simulink model "PD_gravity"  (R2024b)
settings: Solver=ode3  StartTime=0.0  StopTime=inf  FixedStep=0.001  RelTol=1e-3
values from neighbouring files (symbols this model uses):
  p = zeros(60,1)    [UR5e_init.m]
  q0 = zeros(6,1)    [UR5e_init.m]
libraries: robotsim3dlib x1, sim3dlib x1
settings Model: Creator=feder  LastModifiedBy=feder

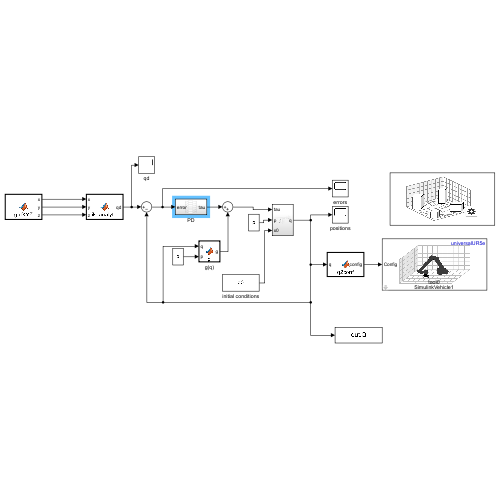
[thumbnail: Simulink's stored preview of the top-level diagram]
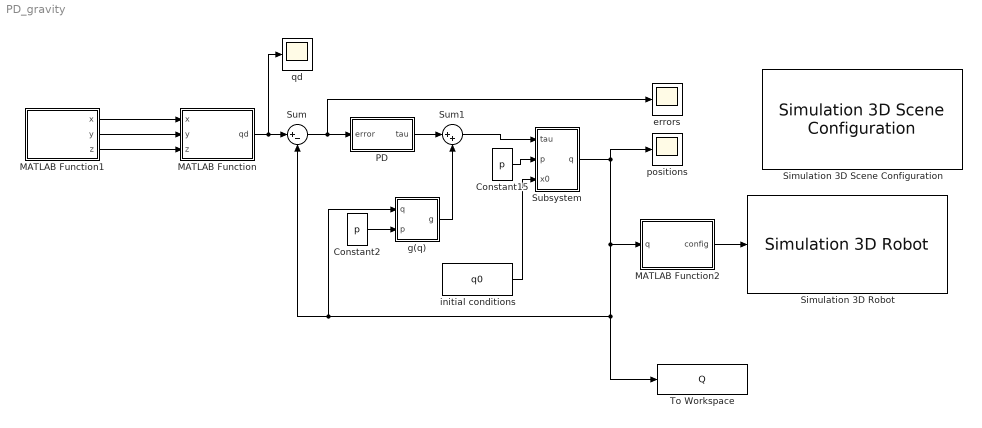
== system PD_gravity ==
  Constant15 : Constant  Value=p
  Constant2 : Constant  Value=p
  MATLAB Function : MATLAB Function  TreatAsAtomicUnit=on
  MATLAB Function1 : MATLAB Function  TreatAsAtomicUnit=on
  MATLAB Function2 : MATLAB Function  TreatAsAtomicUnit=on
  PD : Subsystem
  Simulation 3D Robot : robotsim3dlib/Simulation 3D Robot  actorInputType=Robot Library  RigidBodyTree=universalUR5e  ActorName=SimulinkVehicle1  existActorChekBox=off  initialTrans=[0 0 0]  initialRot=[0 0 0]  initialConfig="[0  0  0  0  0  0]"  EndEffector=tool0  eeOffsetInpChekBox=off  eeTargetTrans=[0 0 0]  eeTargetRot=[0 0 0]  enableRegionGraspChekBox=off  regionGraspInpChekBox=off  eeTargTransDiff=[0.2 0.2 0.2]  eeTargRotDiff=[0 0 0]  inpConfEnbVal=on  inpGraspEnbVal=off  inpTransEnbVal=off  outConfEnbVal=off  outGraspEnbVal=off  outTransEnbVal=off  SampleTime=0.01  ActorType=SimulinkVehicle  ID=1  aMode=6  ActorTag=SimulinkVehicle1  Mesh=RigidBodyTree
  Simulation 3D Scene Configuration : sim3dlib/Simulation 3D Scene Configuration  Priority=0  ProjectFormat=Default Scenes  SceneDesc=Double lane change  ProjectName=C:\Program Files\MATLAB\R2024b\toolbox\shared\sim3d_projects\automotive_project_windows\UE\WindowsNoEditor\VehicleSimulation.exe  ScenePath=/Game/Maps/EmptyScene  EnableOpenDRIVE=off  vehTagList={'Custom';'Scene Origin';'SimulinkVehicle1'}  vehTag=Scene Origin  FreeCameraInitialTranslation=[0, 0, 0]  FreeCameraDefaultInitialTranslation=[-6, 0, 2]  FreeCameraInitialRotation=[0, 0, 0]  FreeCameraDefaultInitialRotation=[0, -15, 0]  OpVisEn=off  Ts=0.001  EnableWindow=on  EnableRemoteAccess=off  EnableWeather=off  SunAzimuth=90  SunAltitude=40.0  EnableGeospatialSun=off  Latitude=0  Longitude=0  Date=2023-01-01  Time=10:30:00  GeoTimeZone=-5.0  SunDaylightSaving=off  wind=1  clouds=10  EnableVolumetricClouds=off  CloudCoverage=0  CloudAltitude=6  fog=0  rain=0  RaindropsEffect=off  SnowDensity=0  EnableGeospatial=off  UseTrueOrigin=off  OriginHeight=200  OriginLatitude=40.744652  OriginLongitude=-73.988864  MapStyle=Aerial  AdditionalAssetIDs=[]  UseAdvancedSunSky=off  SolarTime=11  TimeZone=-5  Day=21  Month=9  Year=2022  UseDaylightSavingTime=on  DSTStartDay=10  DSTStartMonth=3  DSTEndDay=3  DSTEndMonth=11  DSTSwitchHour=2  sensorTag=MainCamera1  sensorId=1  sensorName=MainCamera1  mountLoc=Origin  offsetFlag=off  tmountOffset=[0, 0, 0]  rmountOffset=[0, 0, 0]  HorizontalResolution=1280  VerticalResolution=720  HorizontalFOV=60  mountPoint=[0 0 0]  mountOrientation=[0 0 0]  aMode=6  ID=1  GeoTrigger=Inactive
      settings: LibrarySourceBlock=robotsim3dlib/Simulation 3D Scene Configuration
  Subsystem : Subsystem
  Sum : Sum  Inputs=|+-
  Sum1 : Sum  Inputs=|++
  To Workspace : ToWorkspace  VariableName=Q  SampleTime=0.01
      settings: MaxDataPoints=10
  errors : Scope
  g(q) : MATLAB Function  TreatAsAtomicUnit=on
  initial conditions : Constant  Value=q0
  positions : Scope
  qd : Scope
  wires:
  Constant2/1 -> g(q)/2(p)
  Subsystem/1(q) -> MATLAB Function2/1(q), To Workspace/1, g(q)/1(q), Sum/2, positions/1
  Sum1/1 -> Subsystem/1(tau)
  MATLAB Function/1(qd) -> qd/1, Sum/1
  g(q)/1(g) -> Sum1/2
  initial conditions/1 -> Subsystem/3(x0)
  PD/1(tau) -> Sum1/1
  Constant15/1 -> Subsystem/2(p)
  Sum/1 -> errors/1, PD/1(error)
  MATLAB Function1/1(x) -> MATLAB Function/1(x)
  MATLAB Function1/3(z) -> MATLAB Function/3(z)
  MATLAB Function1/2(y) -> MATLAB Function/2(y)
  MATLAB Function2/1(config) -> Simulation 3D Robot/1

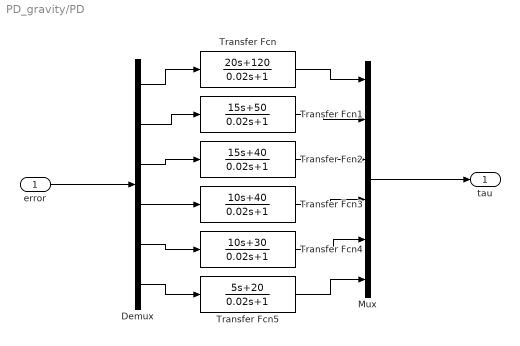
== system PD_gravity/PD ==
  error : Inport  PortDimensions=6
  Demux : Demux  Outputs=6
  Mux : Mux  Inputs=6
  Transfer Fcn : TransferFcn  Numerator=[20 120]  Denominator=[0.02 1]
  Transfer Fcn1 : TransferFcn  Numerator=[15 50]  Denominator=[0.02 1]
  Transfer Fcn2 : TransferFcn  Numerator=[15 40]  Denominator=[0.02 1]
  Transfer Fcn3 : TransferFcn  Numerator=[10 40]  Denominator=[0.02 1]
  Transfer Fcn4 : TransferFcn  Numerator=[10 30]  Denominator=[0.02 1]
  Transfer Fcn5 : TransferFcn  Numerator=[5 20]  Denominator=[0.02 1]
  tau : Outport  PortDimensions=6
  wires:
  Demux/1 -> Transfer Fcn/1
  Demux/2 -> Transfer Fcn1/1
  error/1 -> Demux/1
  Transfer Fcn/1 -> Mux/1
  Transfer Fcn1/1 -> Mux/2
  Mux/1 -> tau/1
  Demux/3 -> Transfer Fcn2/1
  Transfer Fcn2/1 -> Mux/3
  Demux/4 -> Transfer Fcn3/1
  Demux/5 -> Transfer Fcn4/1
  Demux/6 -> Transfer Fcn5/1
  Transfer Fcn3/1 -> Mux/4
  Transfer Fcn4/1 -> Mux/5
  Transfer Fcn5/1 -> Mux/6

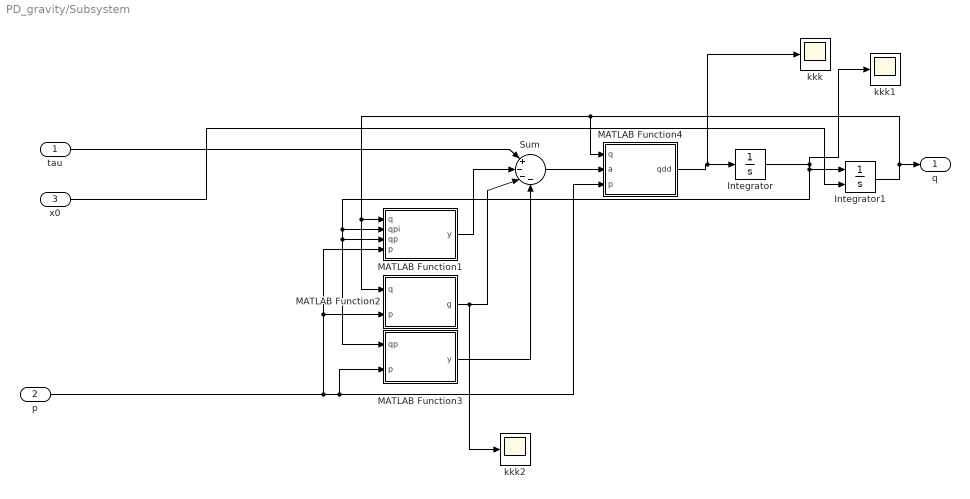
== system PD_gravity/Subsystem ==
  tau : Inport  PortDimensions=6
  p : Inport  Port=2
  x0 : Inport  Port=3
  Integrator : Integrator  InitialCondition=[0.1;0.1;0.1;0.1;0.1;0.1]
  Integrator1 : Integrator  InitialConditionSource=external
  MATLAB Function1 : MATLAB Function  TreatAsAtomicUnit=on
  MATLAB Function2 : MATLAB Function  TreatAsAtomicUnit=on
  MATLAB Function3 : MATLAB Function  TreatAsAtomicUnit=on
  MATLAB Function4 : MATLAB Function  TreatAsAtomicUnit=on
  Sum : Sum  Inputs=|+---
  kkk : Scope
  kkk1 : Scope
  kkk2 : Scope
  q : Outport  PortDimensions=6
  wires:
  MATLAB Function2/1(g) -> kkk2/1, Sum/3
  p/1 -> MATLAB Function1/4(p), MATLAB Function2/2(p), MATLAB Function3/2(p), MATLAB Function4/3(p)
  Integrator1/1 -> MATLAB Function2/1(q), MATLAB Function1/1(q), MATLAB Function4/1(q), q/1
  tau/1 -> Sum/1
  Sum/1 -> MATLAB Function4/2(a)
  Integrator/1 -> Integrator1/1, MATLAB Function1/3(qp), MATLAB Function3/1(qp), MATLAB Function1/2(qpi), kkk1/1
  MATLAB Function1/1(y) -> Sum/2
  MATLAB Function3/1(y) -> Sum/4
  x0/1 -> Integrator1/2
  MATLAB Function4/1(qdd) -> Integrator/1, kkk/1

== matlab function PD_gravity/Subsystem/MATLAB Function1 ==
  data: q input; qpi input; qp input; y output; p input
function y = Cqp(q, qpi, qp, p)
% Cqp_rt_full
% Approssimazione real-time safe di C(q,qd)*qd per UR5e
% Considera tutti gli accoppiamenti principali tra i 6 giunti e i bracci r_i
%
% Input:
% q   [6x1] : posizioni articolari
% qpi [6x1] : velocità articolari (alias di qp, per compatibilità)
% qp  [6x1] : velocità articolari
% p   [60x1]: parametri dinamici UR5e
%
% Output:
% y [6x1] : C(q,qd)*qd approssimato

y = zeros(6,1);

% % ----------------------------
% % Estrazione parametri principali
% % ----------------------------
% m = zeros(6,1);
% r = zeros(6,3);
% 
% for i = 1:6
%     idx = (i-1)*10;
%     m(i) = p(idx+1);            % massa
%     r(i,:) = p(idx+2:idx+4)';   % m*r già incluso in p
% end
% 
% % ----------------------------
% % Termini principali di Coriolis
% % Formula: c_ij = m_j * sin(q_j) * (r_j · r_effect) * qdot_i * qdot_j
% % ----------------------------
% 
% % Giunto 1-2
% y(1) = -m(2) * sin(q(2)) * dot(r(2,:), r(1,:)) * qp(2) * qp(1);
% y(2) =  m(2) * sin(q(2)) * dot(r(2,:), r(1,:)) * qp(1) * qp(2);
% 
% % Giunto 2-3
% y(2) = y(2) - m(3) * sin(q(3)) * dot(r(3,:), r(2,:)) * qp(3) * qp(2);
% y(3) =  m(3) * sin(q(3)) * dot(r(3,:), r(2,:)) * qp(2) * qp(3);
% 
% % Giunto 3-4
% y(3) = y(3) - m(4) * sin(q(4)) * dot(r(4,:), r(3,:)) * qp(4) * qp(3);
% y(4) =  m(4) * sin(q(4)) * dot(r(4,:), r(3,:)) * qp(3) * qp(4);
% 
% % Giunto 4-5
% y(4) = y(4) - m(5) * sin(q(5)) * dot(r(5,:), r(4,:)) * qp(5) * qp(4);
% y(5) =  m(5) * sin(q(5)) * dot(r(5,:), r(4,:)) * qp(4) * qp(5);
% 
% % Giunto 5-6
% y(5) = y(5) - m(6) * sin(q(6)) * dot(r(6,:), r(5,:)) * qp(6) * qp(5);
% y(6) =  m(6) * sin(q(6)) * dot(r(6,:), r(5,:)) * qp(5) * qp(6);

end

== matlab function PD_gravity/g(q) ==
  data: q input; g output; p input
function g = g(q, p)
% g_fullJacobian
% Calcola il termine gravitazionale g(q)
%
% q [6x1]
% p [60x1]

n = 6;
g = zeros(n,1);

g0 = [0; 0; -9.81];   % gravità nel frame base

% --- Estrazione parametri ---
m = zeros(6,1);
r = zeros(6,3);

for i = 1:6
    idx = (i-1)*10;
    m(i) = p(idx+1);
    r(i,:) = p(idx+2:idx+4)' / m(i);
end

% --- DH UR5e ---
L = [0.1625, 0.425, 0.3922, 0.1333, 0.0997, 0.0996];
alpha = [pi/2, 0, 0, pi/2, -pi/2, 0];
d     = [L(1), 0, 0, L(4), L(5), L(6)];
a     = [0, L(2), L(3), 0, 0, 0];

% --- Contributo gravitazionale ---
for iLink = 1:6

    % Cinematica diretta fino al CoM
    T = eye(4);
    for j = 1:iLink
        ct = cos(q(j)); st = sin(q(j));
        ca = cos(alpha(j)); sa = sin(alpha(j));

        A = [ ct  -st*ca  st*sa  a(j)*ct;
              st   ct*ca -ct*sa  a(j)*st;
              0     sa     ca     d(j);
              0     0      0      1 ];
        T = T * A;
    end

    % Posizione CoM nel base frame
    r_i = T(1:3,1:3)*r(iLink,:)' + T(1:3,4);

    % Jacobiana lineare del CoM
    Jv = zeros(3,n);

    Tj = eye(4);
    for j = 1:n
        if j <= iLink
            ct = cos(q(j)); st = sin(q(j));
            ca = cos(alpha(j)); sa = sin(alpha(j));

            A = [ ct  -st*ca  st*sa  a(j)*ct;
                  st   ct*ca -ct*sa  a(j)*st;
                  0     sa     ca     d(j);
                  0     0      0      1 ];
            Tj = Tj * A;

            z = Tj(1:3,3);
            o = Tj(1:3,4);

            Jv(:,j) = cross(z, r_i - o);
        end
    end

    % Contributo gravitazionale del link i
    g = g + Jv' * (m(iLink) * g0);
end

end

== matlab function PD_gravity/Subsystem/MATLAB Function2 ==
  data: q input; g output; p input
function g = g(q, p)
% g_fullJacobian
% Calcola il termine gravitazionale g(q)
%
% q [6x1]
% p [60x1]

n = 6;
g = zeros(n,1);

g0 = [0; 0; -9.81];   % gravità nel frame base

% --- Estrazione parametri ---
m = zeros(6,1);
r = zeros(6,3);

for i = 1:6
    idx = (i-1)*10;
    m(i) = p(idx+1);
    r(i,:) = p(idx+2:idx+4)' / m(i);
end

% --- DH UR5e ---
L = [0.1625, 0.425, 0.3922, 0.1333, 0.0997, 0.0996];
alpha = [pi/2, 0, 0, pi/2, -pi/2, 0];
d     = [L(1), 0, 0, L(4), L(5), L(6)];
a     = [0, L(2), L(3), 0, 0, 0];

% --- Contributo gravitazionale ---
for iLink = 1:6

    % Cinematica diretta fino al CoM
    T = eye(4);
    for j = 1:iLink
        ct = cos(q(j)); st = sin(q(j));
        ca = cos(alpha(j)); sa = sin(alpha(j));

        A = [ ct  -st*ca  st*sa  a(j)*ct;
              st   ct*ca -ct*sa  a(j)*st;
              0     sa     ca     d(j);
              0     0      0      1 ];
        T = T * A;
    end

    % Posizione CoM nel base frame
    r_i = T(1:3,1:3)*r(iLink,:)' + T(1:3,4);

    % Jacobiana lineare del CoM
    Jv = zeros(3,n);

    Tj = eye(4);
    for j = 1:n
        if j <= iLink
            ct = cos(q(j)); st = sin(q(j));
            ca = cos(alpha(j)); sa = sin(alpha(j));

            A = [ ct  -st*ca  st*sa  a(j)*ct;
                  st   ct*ca -ct*sa  a(j)*st;
                  0     sa     ca     d(j);
                  0     0      0      1 ];
            Tj = Tj * A;

            z = Tj(1:3,3);
            o = Tj(1:3,4);

            Jv(:,j) = cross(z, r_i - o);
        end
    end

    % Contributo gravitazionale del link i
    g = g + Jv' * (m(iLink) * g0);
end

end

== matlab function PD_gravity/Subsystem/MATLAB Function3 ==
  data: qp input; y output; p input
function y = fv(qp, p)
% fv
% Attrito viscoso UR5e (6 DOF)
%
% qp [6x1] : velocità articolari
% p  [60x1]: parametri dinamici
%            p(51:56) = coefficienti di attrito viscoso

y = zeros(6,1);

for i = 1:6
    y(i) = p(50 + i) * qp(i);
end

end

== matlab function PD_gravity/Subsystem/MATLAB Function4 ==
  data: q input; a input; qdd output; p input
function qdd = invBa(q, a, p)
% invBa - Calcola qdd = B(q)^(-1) * a per UR5e
%
% INPUTS:
%   q  [6x1]   : variabili di giunto
%   a  [6x1]   : termine noto (tau - C - g - fv)
%   p  [60x1]  : parametri dinamici (6 link × 10)
%
% OUTPUT:
%   qdd [6x1]  : accelerazioni articolari

n = 6;
epsilon = 1e-4; % regolarizzazione finale
B = zeros(n);

% ----------------------------
% Estrazione parametri dinamici
% ----------------------------
m = zeros(6,1);
r = zeros(6,3);
I = zeros(3,3,6);

for i = 1:6
    idx = (i-1)*10;
    m(i) = p(idx+1);
    r(i,:) = p(idx+2:idx+4)' / m(i);
    I(:,:,i) = [ p(idx+5)  p(idx+8)  p(idx+9);
                 p(idx+8)  p(idx+6)  p(idx+10);
                 p(idx+9)  p(idx+10) p(idx+7) ];
end

% ----------------------------
% Parametri DH UR5e
% ----------------------------
L = [0.1625, 0.425, 0.3922, 0.1333, 0.0997, 0.0996];
alpha = [pi/2, 0, 0, pi/2, -pi/2, 0];
d     = [L(1), 0, 0, L(4), L(5), L(6)];
a_dh  = [0, L(2), L(3), 0, 0, 0];

% ----------------------------
% Costruzione matrice di inerzia B(q)
% ----------------------------
for iLink = 1:6

    % Cinematica diretta fino al CoM del link i
    T = eye(4);
    for j = 1:iLink
        ct = cos(q(j)); st = sin(q(j));
        ca = cos(alpha(j)); sa = sin(alpha(j));

        A = [ ct  -st*ca  st*sa  a_dh(j)*ct;
              st   ct*ca -ct*sa  a_dh(j)*st;
              0     sa     ca     d(j);
              0     0      0      1 ];
        T = T * A;
    end

    % Posizione CoM nel frame base
    r_i = T(1:3,1:3)*r(iLink,:)' + T(1:3,4);

    % Jacobiane del CoM
    Jv = zeros(3,n);
    Jw = zeros(3,n);
    Tj = eye(4);

    for j = 1:n
        if j <= iLink
            ct = cos(q(j)); st = sin(q(j));
            ca = cos(alpha(j)); sa = sin(alpha(j));

            A = [ ct  -st*ca  st*sa  a_dh(j)*ct;
                  st   ct*ca -ct*sa  a_dh(j)*st;
                  0     sa     ca     d(j);
                  0     0      0      1 ];
            Tj = Tj * A;

            z = Tj(1:3,3);
            o = Tj(1:3,4);

            Jv(:,j) = cross(z, r_i - o);
            Jw(:,j) = z;
        end
    end

    % Rotazione delle inerzie nel frame base
    R = T(1:3,1:3);
    I_base = R * I(:,:,iLink) * R';
    I_base = 0.5*(I_base + I_base'); % simmetrizzazione numerica

    % Contributo del link i alla matrice di inerzia
    B = B + Jv' * m(iLink) * Jv + Jw' * I_base * Jw;
end

% ----------------------------
% Regolarizzazione finale di B
% ----------------------------
B = B + epsilon*eye(n);

% ----------------------------
% Accelerazioni articolari
% ----------------------------
qdd = B \ a;

end

== matlab function PD_gravity/MATLAB Function ==
  data: x input; qd output; y input; z input
function qd = ik_analytic(x, y, z)
% IK analitica UR5e
% L'end-effector rimane verticale (z verso il basso)
% Configurazione gomito in su

%% Parametri DH UR5e
d1 = 0.1625;
a2 = -0.425;
a3 = -0.3922;
d4 = 0.1333;
d5 = 0.0997;
d6 = 0.0996;

%% Posizione desiderata
pd = [x; y; z];

%% Orientamento desiderato: z verso il basso
R06_des = [0  0 -1;
           0  1  0;
           -1 0  0];

%% Punto del polso
pw = pd - d6 * R06_des(:,3);
xw = pw(1);
yw = pw(2);
zw = pw(3);

%% -------------------------
% Giunto 1
%% -------------------------
q1 = atan2(yw, xw);

%% -------------------------
% Giunti 2 e 3 (piano del braccio, gomito in su)
%% -------------------------
r = sqrt(xw^2 + yw^2);
s = zw - d1;

D = (r^2 + s^2 - a2^2 - a3^2)/(2*a2*a3);
q3 = atan2(-sqrt(1 - D^2), D);  % gomito in su

phi = atan2(s, r);
psi = atan2(a3*sin(q3), a2 + a3*cos(q3));
q2 = phi - psi;

%% -------------------------
% Calcolo R03
%% -------------------------
T01 = trotz(q1)*transl(0,0,d1);
T12 = trotz(q2)*transl(a2,0,0);
T23 = trotz(q3)*transl(a3,0,0);
T03 = T01*T12*T23;
R03 = T03(1:3,1:3);

%% -------------------------
% Giunti polso 4-5-6 (q4, q5, q6)
% Mantiene l'orientamento verticale
%% -------------------------
R36 = R03' * R06_des;

q5 = atan2(sqrt(R36(3,1)^2 + R36(3,2)^2), R36(3,3));
q4 = atan2(R36(2,3), R36(1,3));
q6 = atan2(R36(3,2), -R36(3,1));

%% -------------------------
% Output
%% -------------------------
qd = [q1; q2; q3; q4; q5; q6];

end

== matlab function PD_gravity/MATLAB Function1 ==
  data: x output; y output; z output
function [x, y, z] = getXYZ()
%#codegen
% xyz_out: [1x3] vettore double, output continuo

% Inizializza l’output con tipo e dimensione fissa
x = 0;
y = 0;
z = 0;
% Dichiarazione extrinsic per leggere il workspace base
coder.extrinsic('evalin');

% Leggi le variabili live dal workspace
x_val = evalin('base', 'x');
y_val = evalin('base', 'y');
z_val = evalin('base', 'z');

% Assegna all’output
x = double(x_val);
y = double(y_val);
z = double(z_val);
end

== matlab function PD_gravity/MATLAB Function2 ==
  data: q input; config output
function config = q2conf(q)

config = q(:)';
end
